simulink model "SinglePhasePVGridConnettedArray"  (R2024a)
settings: Solver=VariableStepAuto  StartTime=0.0  StopTime=0.1  RelTol=1e-3
libraries: spsMosfetLib x12, spsSeriesRLCBranchLib x12, spsCurrentMeasurementLib x6, spsFirstOrderFilterLib x6, slpidlib x6, simulink x6, spsVoltageMeasurementLib x6, spsACVoltageSourceLib x3, spsAlphaBetaZerotodq0Lib x3, spsPVArrayLib x3, spspowerguiLib x3
settings Model: Creator=Akbar  LastModifiedBy=Akbar
settings OptimizationCC: ReuseModelBlockBuffer=off
settings RTWCC: GPUComputeCapability=3.5

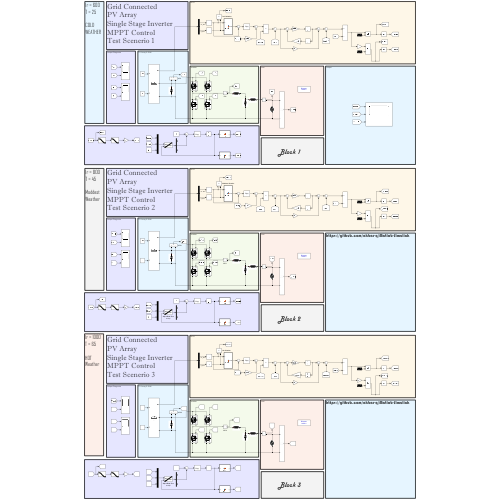
[thumbnail: Simulink's stored preview of the top-level diagram]
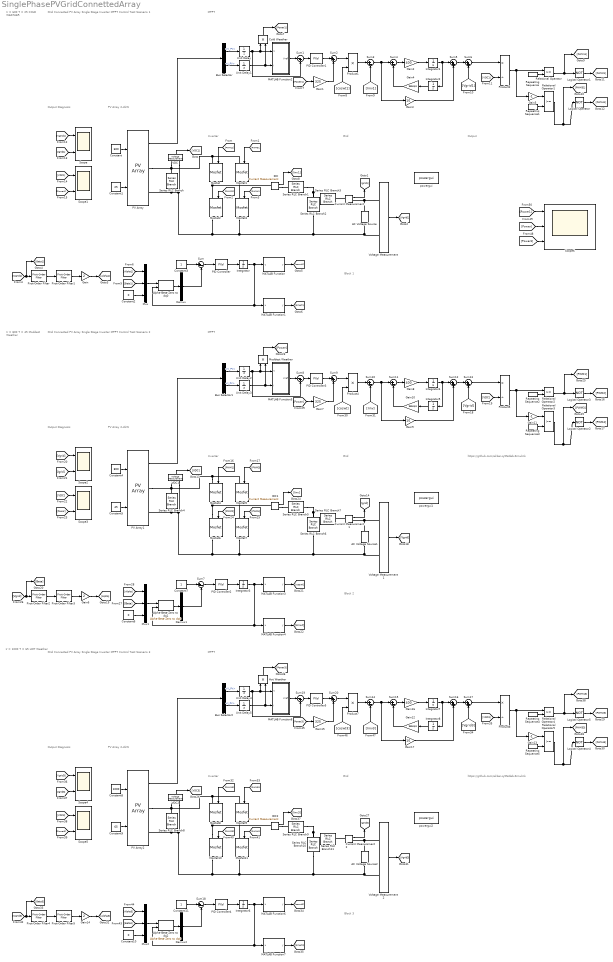
== system SinglePhasePVGridConnettedArray ==
  note: Output
  note: Ir = 600
      | T = 25
      |
      | COLD
      | WEATHER
  note: Grid Connected
      | PV Array
      | Single Stage Inverter
      | MPPT Control
      | Test Scenerio 1
  note: Block 1
  note: Grid
  note: Inverter
  note: PV Array 2-3kW
  note: MPPT
  note: Output Diagnosis
  note: Ir = 800
      | T = 45
      |
      | Moddest
      | Weather
  note: Grid Connected
      | PV Array
      | Single Stage Inverter
      | MPPT Control
      | Test Scenerio 2
  note: Inverter
  note: Grid
  note: PV Array 2-3kW
  note: Block 2
  note: Output Diagnosis
  note: MPPT
  note: Block 3
  note: PV Array 2-3kW
  note: Grid
  note: MPPT
  note: Output Diagnosis
  note: Ir = 1000
      | T = 65
      |
      | HOT
      | Weather
  note: Inverter
  note: Grid Connected
      | PV Array
      | Single Stage Inverter
      | MPPT Control
      | Test Scenerio 3
  note: https://github.com/akbar-q/Matlab-Simulink
  note: https://github.com/akbar-q/Matlab-Simulink
  AC Voltage Source : spsACVoltageSourceLib/AC Voltage Source  Amplitude=325  Phase=0  Frequency=50  SampleTime=0  Measurements=None  BusType=swing  Pref=10e3  Qref=0  Qmin=-inf  Qmax=+inf
  AC Voltage Source1 : spsACVoltageSourceLib/AC Voltage Source  Amplitude=325  Phase=0  Frequency=50  SampleTime=0  Measurements=None  BusType=swing  Pref=10e3  Qref=0  Qmin=-inf  Qmax=+inf
  AC Voltage Source2 : spsACVoltageSourceLib/AC Voltage Source  Amplitude=325  Phase=0  Frequency=50  SampleTime=0  Measurements=None  BusType=swing  Pref=10e3  Qref=0  Qmin=-inf  Qmax=+inf
  Alpha-Beta-Zero to dq0 : spsAlphaBetaZerotodq0Lib/Alpha-Beta-Zero to dq0  Alignment=90 degrees behind phase A axis
  Alpha-Beta-Zero to dq1 : spsAlphaBetaZerotodq0Lib/Alpha-Beta-Zero to dq0  Alignment=90 degrees behind phase A axis
  Alpha-Beta-Zero to dq2 : spsAlphaBetaZerotodq0Lib/Alpha-Beta-Zero to dq0  Alignment=90 degrees behind phase A axis
  Bus Selector : BusSelector  OutputSignals=V_PV,I_PV
  Bus Selector1 : BusSelector  OutputSignals=V_PV,I_PV
  Bus Selector2 : BusSelector  OutputSignals=V_PV,I_PV
  Cold Weather : Product
  Constant : Constant  Value=600
  Constant1 : Constant  Value=25
  Constant10 : Constant  Value=0
  Constant11 : Constant
  Constant2 : Constant  Value=0
  Constant3 : Constant
  Constant4 : Constant  Value=800
  Constant5 : Constant  Value=45
  Constant6 : Constant  Value=0
  Constant7 : Constant
  Constant8 : Constant  Value=1000
  Constant9 : Constant  Value=65
  Current Measurement : spsCurrentMeasurementLib/Current Measurement  PhasorSimulation=off  OutputType=Complex  PSBequivalent=0
  Current Measurement1 : spsCurrentMeasurementLib/Current Measurement  PhasorSimulation=off  OutputType=Complex  PSBequivalent=0
  Current Measurement2 : spsCurrentMeasurementLib/Current Measurement  PhasorSimulation=off  OutputType=Complex  PSBequivalent=0
  Demux : Demux  Outputs=3
  Demux1 : Demux  Outputs=3
  Demux2 : Demux  Outputs=3
  First-Order Filter{,1..5} (6 alike) : spsFirstOrderFilterLib/First-Order Filter  FilterType=Lowpass  Tc=1/(2*pi*50)  Ts=0  Initialize=off  Vac_Init=[0, 0, 60]  Vdc_Init=0  PlotResponse=off  FreqRange="[0,  200,  1]"
  Gain : Gain  Gain=2
  Gain1 : Gain  Gain=325
  Gain10 : Gain  Gain=986.8/4
  Gain11 : Gain  Gain=-1
  Gain12 : Gain  Gain=986.8/4
  Gain13 : Gain  Gain=-1
  Gain14 : Gain  Gain=2
  Gain15 : Gain  Gain=325
  Gain16 : Gain  Gain=400
  Gain17 : Gain  Gain=10
  Gain2 : Gain  Gain=400
  Gain3 : Gain  Gain=10
  Gain4 : Gain  Gain=986.8/4
  Gain5 : Gain  Gain=-1
  Gain6 : Gain  Gain=2
  Gain7 : Gain  Gain=325
  Gain8 : Gain  Gain=400
  Gain9 : Gain  Gain=10
  Hot Weather : Product
  IDC : spsCurrentMeasurementLib/Current Measurement  PhasorSimulation=off  OutputType=Complex  PSBequivalent=0
  IDC1 : spsCurrentMeasurementLib/Current Measurement  PhasorSimulation=off  OutputType=Complex  PSBequivalent=0
  IDC2 : spsCurrentMeasurementLib/Current Measurement  PhasorSimulation=off  OutputType=Complex  PSBequivalent=0
  Integrator{,1..8} (9 alike) : Integrator
  Logical Operator{,1..5} (6 alike) : Logic  Operator=NOT  AllPortsSameDT=off  OutDataTypeStr=boolean
  MATLAB Function : MATLAB Function  TreatAsAtomicUnit=on
  MATLAB Function1 : MATLAB Function  TreatAsAtomicUnit=on
  MATLAB Function2 : MATLAB Function  TreatAsAtomicUnit=on
  MATLAB Function3 : MATLAB Function  TreatAsAtomicUnit=on
  MATLAB Function4 : MATLAB Function  TreatAsAtomicUnit=on
  MATLAB Function5 : MATLAB Function  TreatAsAtomicUnit=on
  MATLAB Function6 : MATLAB Function  TreatAsAtomicUnit=on
  MATLAB Function7 : MATLAB Function  TreatAsAtomicUnit=on
  MATLAB Function8 : MATLAB Function  TreatAsAtomicUnit=on
  Moddest Weather : Product
  Mosfet{,1..11} (12 alike) : spsMosfetLib/Mosfet  Ron=0.1  Lon=0  Rd=0.01  Vfd=0  IC=0  Rs=1e5  Cs=inf  Measurements=on
  Mux : Mux  Inputs=3
  Mux1 : Mux  Inputs=3
  Mux2 : Mux  Inputs=3
  PID Controller : slpidlib/PID Controller  Controller=PI  Form=Parallel  TimeDomain=Continuous-time  UseExternalTs=off  SampleTime=-1  IntegratorMethod=Forward Euler  FilterMethod=Forward Euler  ControllerParametersSource=internal  P=10  I=5000  UseKiTs=off  D=0  UseExternalDerivativeSource=off  N=100  UseFilter=on  TunerSelectOption=Transfer Function Based (PID Tuner App)  InitialConditionSource=internal  InitialConditionForIntegrator=0  InitialConditionForFilter=0  DifferentiatorICPrevScaledInput=0  ExternalReset=none  TrackingMode=off  Kt=1  LimitOutput=off  SatLimitsSource=internal  UpperSaturationLimit=inf  LowerSaturationLimit=-inf  LinearizeAsGain=on  AntiWindupMode=none  Kb=1  LimitIntegrator=off  UpperIntegratorSaturationLimit=inf  LowerIntegratorSaturationLimit=-inf  POutMin=[]  POutMax=[]  IOutMin=[]  IOutMax=[]  DOutMin=[]  DOutMax=[]  NOutMin=[]  NOutMax=[]  SumOutMin=[]  SumOutMax=[]  SaturationOutMin=[]  SaturationOutMax=[]  PParamMin=[]  PParamMax=[]  IParamMin=[]  IParamMax=[]  DParamMin=[]  DParamMax=[]  NParamMin=[]  NParamMax=[]  KbParamMin=[]  KbParamMax=[]  KtParamMin=[]  KtParamMax=[]  KbOutMin=[]  KbOutMax=[]  KtOutMin=[]  KtOutMax=[]  IntegratorOutMin=[]  IntegratorOutMax=[]  FilterOutMin=[]  FilterOutMax=[]  SumI1OutMin=[]  SumI1OutMax=[]  SumI2OutMin=[]  SumI2OutMax=[]  SumI3OutMin=[]  SumI3OutMax=[]  SumI4OutMin=[]  SumI4OutMax=[]  SumDOutMin=[]  SumDOutMax=[]  DifferentiatorOutMin=[]  DifferentiatorOutMax=[]  FilterDiffOutCoefMin=[]  FilterDiffOutCoefMax=[]  ReciprocalOutMin=[]  ReciprocalOutMax=[]  SumDenOutMin=[]  SumDenOutMax=[]  SumNumOutMin=[]  SumNumOutMax=[]  DivideOutMin=[]  DivideOutMax=[]  UdiffTsProdOutMin=[]  UdiffTsProdOutMax=[]  NTsProdOutMin=[]  NTsProdOutMax=[]  UintegralTsProdOutMin=[]  UintegralTsProdOutMax=[]  UngainTsProdOutMin=[]  UngainTsProdOutMax=[]  ClampingZeroOutDataTypeStr=Inherit: Inherit via back propagation  ClampingZeroOutMin=[]  ClampingZeroOutMax=[]  FilterDenConstantOutDataTypeStr=Inherit: Inherit via back propagation  FilterDenConstantOutMin=[]  FilterDenConstantOutMax=[]  PCopyOutDataTypeStr=Inherit: Inherit via back propagation  PCopyOutMin=[]  PCopyOutMax=[]  NCopyOutDataTypeStr=Inherit: Inherit via back propagation  NCopyOutMin=[]  NCopyOutMax=[]  IntegratorContinuousStateAttributes=''  IntegratorStateMustResolveToSignalObject=off  IntegratorRTWStateStorageClass=Auto  FilterContinuousStateAttributes=''  FilterStateMustResolveToSignalObject=off  FilterRTWStateStorageClass=Auto  ParallelPVariant=InternalParameters  IdealPVariant=Disabled  IVariant=InternalParameters  DVariant=Disabled  IntegratorVariant=Continuous  SatVariant=Disabled  AWVariant=Passthrough  PCopyVariant=Disabled  TRVariant=Disabled  FdbkBlocksVariant=Forward  IdealPFdbkVariant=Disabled  SatFdbkVariant=Disabled  DerivativeFilterVariant=Disabled  NVariant=Disabled  NCopyVariant=Disabled_SignalSpec  FilterICVariant=Disabled  IntegratorICVariant=InternalICs  ExternalResetVariant=Disabled  TRSumVariant=Passthrough  SumFdbkVariant=Disabled  SumVariant=Sum_PI  TsampFilterVariant=InternalTs  TsampNgainVariant=Passthrough  TsampIntegralVariant=Disabled_SignalSpec  ExternalSaturationOutDataTypeStr=Inherit: Same as second input  DerivativeSourceVariant=Disabled
  PID Controller1 : slpidlib/PID Controller  Controller=PI  Form=Parallel  TimeDomain=Continuous-time  UseExternalTs=off  SampleTime=-1  IntegratorMethod=Forward Euler  FilterMethod=Forward Euler  ControllerParametersSource=internal  P=0.075  I=0.075  UseKiTs=off  D=0  UseExternalDerivativeSource=off  N=100  UseFilter=on  TunerSelectOption=Transfer Function Based (PID Tuner App)  InitialConditionSource=internal  InitialConditionForIntegrator=0  InitialConditionForFilter=0  DifferentiatorICPrevScaledInput=0  ExternalReset=none  TrackingMode=off  Kt=1  LimitOutput=off  SatLimitsSource=internal  UpperSaturationLimit=inf  LowerSaturationLimit=-inf  LinearizeAsGain=on  AntiWindupMode=none  Kb=1  LimitIntegrator=off  UpperIntegratorSaturationLimit=inf  LowerIntegratorSaturationLimit=-inf  POutMin=[]  POutMax=[]  IOutMin=[]  IOutMax=[]  DOutMin=[]  DOutMax=[]  NOutMin=[]  NOutMax=[]  SumOutMin=[]  SumOutMax=[]  SaturationOutMin=[]  SaturationOutMax=[]  PParamMin=[]  PParamMax=[]  IParamMin=[]  IParamMax=[]  DParamMin=[]  DParamMax=[]  NParamMin=[]  NParamMax=[]  KbParamMin=[]  KbParamMax=[]  KtParamMin=[]  KtParamMax=[]  KbOutMin=[]  KbOutMax=[]  KtOutMin=[]  KtOutMax=[]  IntegratorOutMin=[]  IntegratorOutMax=[]  FilterOutMin=[]  FilterOutMax=[]  SumI1OutMin=[]  SumI1OutMax=[]  SumI2OutMin=[]  SumI2OutMax=[]  SumI3OutMin=[]  SumI3OutMax=[]  SumI4OutMin=[]  SumI4OutMax=[]  SumDOutMin=[]  SumDOutMax=[]  DifferentiatorOutMin=[]  DifferentiatorOutMax=[]  FilterDiffOutCoefMin=[]  FilterDiffOutCoefMax=[]  ReciprocalOutMin=[]  ReciprocalOutMax=[]  SumDenOutMin=[]  SumDenOutMax=[]  SumNumOutMin=[]  SumNumOutMax=[]  DivideOutMin=[]  DivideOutMax=[]  UdiffTsProdOutMin=[]  UdiffTsProdOutMax=[]  NTsProdOutMin=[]  NTsProdOutMax=[]  UintegralTsProdOutMin=[]  UintegralTsProdOutMax=[]  UngainTsProdOutMin=[]  UngainTsProdOutMax=[]  ClampingZeroOutDataTypeStr=Inherit: Inherit via back propagation  ClampingZeroOutMin=[]  ClampingZeroOutMax=[]  FilterDenConstantOutDataTypeStr=Inherit: Inherit via back propagation  FilterDenConstantOutMin=[]  FilterDenConstantOutMax=[]  PCopyOutDataTypeStr=Inherit: Inherit via back propagation  PCopyOutMin=[]  PCopyOutMax=[]  NCopyOutDataTypeStr=Inherit: Inherit via back propagation  NCopyOutMin=[]  NCopyOutMax=[]  IntegratorContinuousStateAttributes=''  IntegratorStateMustResolveToSignalObject=off  IntegratorRTWStateStorageClass=Auto  FilterContinuousStateAttributes=''  FilterStateMustResolveToSignalObject=off  FilterRTWStateStorageClass=Auto  ParallelPVariant=InternalParameters  IdealPVariant=Disabled  IVariant=InternalParameters  DVariant=Disabled  IntegratorVariant=Continuous  SatVariant=Disabled  AWVariant=Passthrough  PCopyVariant=Disabled  TRVariant=Disabled  FdbkBlocksVariant=Forward  IdealPFdbkVariant=Disabled  SatFdbkVariant=Disabled  DerivativeFilterVariant=Disabled  NVariant=Disabled  NCopyVariant=Disabled_SignalSpec  FilterICVariant=Disabled  IntegratorICVariant=InternalICs  ExternalResetVariant=Disabled  TRSumVariant=Passthrough  SumFdbkVariant=Disabled  SumVariant=Sum_PI  TsampFilterVariant=InternalTs  TsampNgainVariant=Passthrough  TsampIntegralVariant=Disabled_SignalSpec  ExternalSaturationOutDataTypeStr=Inherit: Same as second input  DerivativeSourceVariant=Disabled
  PID Controller2 : slpidlib/PID Controller  Controller=PI  Form=Parallel  TimeDomain=Continuous-time  UseExternalTs=off  SampleTime=-1  IntegratorMethod=Forward Euler  FilterMethod=Forward Euler  ControllerParametersSource=internal  P=10  I=5000  UseKiTs=off  D=0  UseExternalDerivativeSource=off  N=100  UseFilter=on  TunerSelectOption=Transfer Function Based (PID Tuner App)  InitialConditionSource=internal  InitialConditionForIntegrator=0  InitialConditionForFilter=0  DifferentiatorICPrevScaledInput=0  ExternalReset=none  TrackingMode=off  Kt=1  LimitOutput=off  SatLimitsSource=internal  UpperSaturationLimit=inf  LowerSaturationLimit=-inf  LinearizeAsGain=on  AntiWindupMode=none  Kb=1  LimitIntegrator=off  UpperIntegratorSaturationLimit=inf  LowerIntegratorSaturationLimit=-inf  POutMin=[]  POutMax=[]  IOutMin=[]  IOutMax=[]  DOutMin=[]  DOutMax=[]  NOutMin=[]  NOutMax=[]  SumOutMin=[]  SumOutMax=[]  SaturationOutMin=[]  SaturationOutMax=[]  PParamMin=[]  PParamMax=[]  IParamMin=[]  IParamMax=[]  DParamMin=[]  DParamMax=[]  NParamMin=[]  NParamMax=[]  KbParamMin=[]  KbParamMax=[]  KtParamMin=[]  KtParamMax=[]  KbOutMin=[]  KbOutMax=[]  KtOutMin=[]  KtOutMax=[]  IntegratorOutMin=[]  IntegratorOutMax=[]  FilterOutMin=[]  FilterOutMax=[]  SumI1OutMin=[]  SumI1OutMax=[]  SumI2OutMin=[]  SumI2OutMax=[]  SumI3OutMin=[]  SumI3OutMax=[]  SumI4OutMin=[]  SumI4OutMax=[]  SumDOutMin=[]  SumDOutMax=[]  DifferentiatorOutMin=[]  DifferentiatorOutMax=[]  FilterDiffOutCoefMin=[]  FilterDiffOutCoefMax=[]  ReciprocalOutMin=[]  ReciprocalOutMax=[]  SumDenOutMin=[]  SumDenOutMax=[]  SumNumOutMin=[]  SumNumOutMax=[]  DivideOutMin=[]  DivideOutMax=[]  UdiffTsProdOutMin=[]  UdiffTsProdOutMax=[]  NTsProdOutMin=[]  NTsProdOutMax=[]  UintegralTsProdOutMin=[]  UintegralTsProdOutMax=[]  UngainTsProdOutMin=[]  UngainTsProdOutMax=[]  ClampingZeroOutDataTypeStr=Inherit: Inherit via back propagation  ClampingZeroOutMin=[]  ClampingZeroOutMax=[]  FilterDenConstantOutDataTypeStr=Inherit: Inherit via back propagation  FilterDenConstantOutMin=[]  FilterDenConstantOutMax=[]  PCopyOutDataTypeStr=Inherit: Inherit via back propagation  PCopyOutMin=[]  PCopyOutMax=[]  NCopyOutDataTypeStr=Inherit: Inherit via back propagation  NCopyOutMin=[]  NCopyOutMax=[]  IntegratorContinuousStateAttributes=''  IntegratorStateMustResolveToSignalObject=off  IntegratorRTWStateStorageClass=Auto  FilterContinuousStateAttributes=''  FilterStateMustResolveToSignalObject=off  FilterRTWStateStorageClass=Auto  ParallelPVariant=InternalParameters  IdealPVariant=Disabled  IVariant=InternalParameters  DVariant=Disabled  IntegratorVariant=Continuous  SatVariant=Disabled  AWVariant=Passthrough  PCopyVariant=Disabled  TRVariant=Disabled  FdbkBlocksVariant=Forward  IdealPFdbkVariant=Disabled  SatFdbkVariant=Disabled  DerivativeFilterVariant=Disabled  NVariant=Disabled  NCopyVariant=Disabled_SignalSpec  FilterICVariant=Disabled  IntegratorICVariant=InternalICs  ExternalResetVariant=Disabled  TRSumVariant=Passthrough  SumFdbkVariant=Disabled  SumVariant=Sum_PI  TsampFilterVariant=InternalTs  TsampNgainVariant=Passthrough  TsampIntegralVariant=Disabled_SignalSpec  ExternalSaturationOutDataTypeStr=Inherit: Same as second input  DerivativeSourceVariant=Disabled
  PID Controller3 : slpidlib/PID Controller  Controller=PI  Form=Parallel  TimeDomain=Continuous-time  UseExternalTs=off  SampleTime=-1  IntegratorMethod=Forward Euler  FilterMethod=Forward Euler  ControllerParametersSource=internal  P=0.075  I=0.075  UseKiTs=off  D=0  UseExternalDerivativeSource=off  N=100  UseFilter=on  TunerSelectOption=Transfer Function Based (PID Tuner App)  InitialConditionSource=internal  InitialConditionForIntegrator=0  InitialConditionForFilter=0  DifferentiatorICPrevScaledInput=0  ExternalReset=none  TrackingMode=off  Kt=1  LimitOutput=off  SatLimitsSource=internal  UpperSaturationLimit=inf  LowerSaturationLimit=-inf  LinearizeAsGain=on  AntiWindupMode=none  Kb=1  LimitIntegrator=off  UpperIntegratorSaturationLimit=inf  LowerIntegratorSaturationLimit=-inf  POutMin=[]  POutMax=[]  IOutMin=[]  IOutMax=[]  DOutMin=[]  DOutMax=[]  NOutMin=[]  NOutMax=[]  SumOutMin=[]  SumOutMax=[]  SaturationOutMin=[]  SaturationOutMax=[]  PParamMin=[]  PParamMax=[]  IParamMin=[]  IParamMax=[]  DParamMin=[]  DParamMax=[]  NParamMin=[]  NParamMax=[]  KbParamMin=[]  KbParamMax=[]  KtParamMin=[]  KtParamMax=[]  KbOutMin=[]  KbOutMax=[]  KtOutMin=[]  KtOutMax=[]  IntegratorOutMin=[]  IntegratorOutMax=[]  FilterOutMin=[]  FilterOutMax=[]  SumI1OutMin=[]  SumI1OutMax=[]  SumI2OutMin=[]  SumI2OutMax=[]  SumI3OutMin=[]  SumI3OutMax=[]  SumI4OutMin=[]  SumI4OutMax=[]  SumDOutMin=[]  SumDOutMax=[]  DifferentiatorOutMin=[]  DifferentiatorOutMax=[]  FilterDiffOutCoefMin=[]  FilterDiffOutCoefMax=[]  ReciprocalOutMin=[]  ReciprocalOutMax=[]  SumDenOutMin=[]  SumDenOutMax=[]  SumNumOutMin=[]  SumNumOutMax=[]  DivideOutMin=[]  DivideOutMax=[]  UdiffTsProdOutMin=[]  UdiffTsProdOutMax=[]  NTsProdOutMin=[]  NTsProdOutMax=[]  UintegralTsProdOutMin=[]  UintegralTsProdOutMax=[]  UngainTsProdOutMin=[]  UngainTsProdOutMax=[]  ClampingZeroOutDataTypeStr=Inherit: Inherit via back propagation  ClampingZeroOutMin=[]  ClampingZeroOutMax=[]  FilterDenConstantOutDataTypeStr=Inherit: Inherit via back propagation  FilterDenConstantOutMin=[]  FilterDenConstantOutMax=[]  PCopyOutDataTypeStr=Inherit: Inherit via back propagation  PCopyOutMin=[]  PCopyOutMax=[]  NCopyOutDataTypeStr=Inherit: Inherit via back propagation  NCopyOutMin=[]  NCopyOutMax=[]  IntegratorContinuousStateAttributes=''  IntegratorStateMustResolveToSignalObject=off  IntegratorRTWStateStorageClass=Auto  FilterContinuousStateAttributes=''  FilterStateMustResolveToSignalObject=off  FilterRTWStateStorageClass=Auto  ParallelPVariant=InternalParameters  IdealPVariant=Disabled  IVariant=InternalParameters  DVariant=Disabled  IntegratorVariant=Continuous  SatVariant=Disabled  AWVariant=Passthrough  PCopyVariant=Disabled  TRVariant=Disabled  FdbkBlocksVariant=Forward  IdealPFdbkVariant=Disabled  SatFdbkVariant=Disabled  DerivativeFilterVariant=Disabled  NVariant=Disabled  NCopyVariant=Disabled_SignalSpec  FilterICVariant=Disabled  IntegratorICVariant=InternalICs  ExternalResetVariant=Disabled  TRSumVariant=Passthrough  SumFdbkVariant=Disabled  SumVariant=Sum_PI  TsampFilterVariant=InternalTs  TsampNgainVariant=Passthrough  TsampIntegralVariant=Disabled_SignalSpec  ExternalSaturationOutDataTypeStr=Inherit: Same as second input  DerivativeSourceVariant=Disabled
  PID Controller4 : slpidlib/PID Controller  Controller=PI  Form=Parallel  TimeDomain=Continuous-time  UseExternalTs=off  SampleTime=-1  IntegratorMethod=Forward Euler  FilterMethod=Forward Euler  ControllerParametersSource=internal  P=10  I=5000  UseKiTs=off  D=0  UseExternalDerivativeSource=off  N=100  UseFilter=on  TunerSelectOption=Transfer Function Based (PID Tuner App)  InitialConditionSource=internal  InitialConditionForIntegrator=0  InitialConditionForFilter=0  DifferentiatorICPrevScaledInput=0  ExternalReset=none  TrackingMode=off  Kt=1  LimitOutput=off  SatLimitsSource=internal  UpperSaturationLimit=inf  LowerSaturationLimit=-inf  LinearizeAsGain=on  AntiWindupMode=none  Kb=1  LimitIntegrator=off  UpperIntegratorSaturationLimit=inf  LowerIntegratorSaturationLimit=-inf  POutMin=[]  POutMax=[]  IOutMin=[]  IOutMax=[]  DOutMin=[]  DOutMax=[]  NOutMin=[]  NOutMax=[]  SumOutMin=[]  SumOutMax=[]  SaturationOutMin=[]  SaturationOutMax=[]  PParamMin=[]  PParamMax=[]  IParamMin=[]  IParamMax=[]  DParamMin=[]  DParamMax=[]  NParamMin=[]  NParamMax=[]  KbParamMin=[]  KbParamMax=[]  KtParamMin=[]  KtParamMax=[]  KbOutMin=[]  KbOutMax=[]  KtOutMin=[]  KtOutMax=[]  IntegratorOutMin=[]  IntegratorOutMax=[]  FilterOutMin=[]  FilterOutMax=[]  SumI1OutMin=[]  SumI1OutMax=[]  SumI2OutMin=[]  SumI2OutMax=[]  SumI3OutMin=[]  SumI3OutMax=[]  SumI4OutMin=[]  SumI4OutMax=[]  SumDOutMin=[]  SumDOutMax=[]  DifferentiatorOutMin=[]  DifferentiatorOutMax=[]  FilterDiffOutCoefMin=[]  FilterDiffOutCoefMax=[]  ReciprocalOutMin=[]  ReciprocalOutMax=[]  SumDenOutMin=[]  SumDenOutMax=[]  SumNumOutMin=[]  SumNumOutMax=[]  DivideOutMin=[]  DivideOutMax=[]  UdiffTsProdOutMin=[]  UdiffTsProdOutMax=[]  NTsProdOutMin=[]  NTsProdOutMax=[]  UintegralTsProdOutMin=[]  UintegralTsProdOutMax=[]  UngainTsProdOutMin=[]  UngainTsProdOutMax=[]  ClampingZeroOutDataTypeStr=Inherit: Inherit via back propagation  ClampingZeroOutMin=[]  ClampingZeroOutMax=[]  FilterDenConstantOutDataTypeStr=Inherit: Inherit via back propagation  FilterDenConstantOutMin=[]  FilterDenConstantOutMax=[]  PCopyOutDataTypeStr=Inherit: Inherit via back propagation  PCopyOutMin=[]  PCopyOutMax=[]  NCopyOutDataTypeStr=Inherit: Inherit via back propagation  NCopyOutMin=[]  NCopyOutMax=[]  IntegratorContinuousStateAttributes=''  IntegratorStateMustResolveToSignalObject=off  IntegratorRTWStateStorageClass=Auto  FilterContinuousStateAttributes=''  FilterStateMustResolveToSignalObject=off  FilterRTWStateStorageClass=Auto  ParallelPVariant=InternalParameters  IdealPVariant=Disabled  IVariant=InternalParameters  DVariant=Disabled  IntegratorVariant=Continuous  SatVariant=Disabled  AWVariant=Passthrough  PCopyVariant=Disabled  TRVariant=Disabled  FdbkBlocksVariant=Forward  IdealPFdbkVariant=Disabled  SatFdbkVariant=Disabled  DerivativeFilterVariant=Disabled  NVariant=Disabled  NCopyVariant=Disabled_SignalSpec  FilterICVariant=Disabled  IntegratorICVariant=InternalICs  ExternalResetVariant=Disabled  TRSumVariant=Passthrough  SumFdbkVariant=Disabled  SumVariant=Sum_PI  TsampFilterVariant=InternalTs  TsampNgainVariant=Passthrough  TsampIntegralVariant=Disabled_SignalSpec  ExternalSaturationOutDataTypeStr=Inherit: Same as second input  DerivativeSourceVariant=Disabled
  PID Controller5 : slpidlib/PID Controller  Controller=PI  Form=Parallel  TimeDomain=Continuous-time  UseExternalTs=off  SampleTime=-1  IntegratorMethod=Forward Euler  FilterMethod=Forward Euler  ControllerParametersSource=internal  P=0.075  I=0.075  UseKiTs=off  D=0  UseExternalDerivativeSource=off  N=100  UseFilter=on  TunerSelectOption=Transfer Function Based (PID Tuner App)  InitialConditionSource=internal  InitialConditionForIntegrator=0  InitialConditionForFilter=0  DifferentiatorICPrevScaledInput=0  ExternalReset=none  TrackingMode=off  Kt=1  LimitOutput=off  SatLimitsSource=internal  UpperSaturationLimit=inf  LowerSaturationLimit=-inf  LinearizeAsGain=on  AntiWindupMode=none  Kb=1  LimitIntegrator=off  UpperIntegratorSaturationLimit=inf  LowerIntegratorSaturationLimit=-inf  POutMin=[]  POutMax=[]  IOutMin=[]  IOutMax=[]  DOutMin=[]  DOutMax=[]  NOutMin=[]  NOutMax=[]  SumOutMin=[]  SumOutMax=[]  SaturationOutMin=[]  SaturationOutMax=[]  PParamMin=[]  PParamMax=[]  IParamMin=[]  IParamMax=[]  DParamMin=[]  DParamMax=[]  NParamMin=[]  NParamMax=[]  KbParamMin=[]  KbParamMax=[]  KtParamMin=[]  KtParamMax=[]  KbOutMin=[]  KbOutMax=[]  KtOutMin=[]  KtOutMax=[]  IntegratorOutMin=[]  IntegratorOutMax=[]  FilterOutMin=[]  FilterOutMax=[]  SumI1OutMin=[]  SumI1OutMax=[]  SumI2OutMin=[]  SumI2OutMax=[]  SumI3OutMin=[]  SumI3OutMax=[]  SumI4OutMin=[]  SumI4OutMax=[]  SumDOutMin=[]  SumDOutMax=[]  DifferentiatorOutMin=[]  DifferentiatorOutMax=[]  FilterDiffOutCoefMin=[]  FilterDiffOutCoefMax=[]  ReciprocalOutMin=[]  ReciprocalOutMax=[]  SumDenOutMin=[]  SumDenOutMax=[]  SumNumOutMin=[]  SumNumOutMax=[]  DivideOutMin=[]  DivideOutMax=[]  UdiffTsProdOutMin=[]  UdiffTsProdOutMax=[]  NTsProdOutMin=[]  NTsProdOutMax=[]  UintegralTsProdOutMin=[]  UintegralTsProdOutMax=[]  UngainTsProdOutMin=[]  UngainTsProdOutMax=[]  ClampingZeroOutDataTypeStr=Inherit: Inherit via back propagation  ClampingZeroOutMin=[]  ClampingZeroOutMax=[]  FilterDenConstantOutDataTypeStr=Inherit: Inherit via back propagation  FilterDenConstantOutMin=[]  FilterDenConstantOutMax=[]  PCopyOutDataTypeStr=Inherit: Inherit via back propagation  PCopyOutMin=[]  PCopyOutMax=[]  NCopyOutDataTypeStr=Inherit: Inherit via back propagation  NCopyOutMin=[]  NCopyOutMax=[]  IntegratorContinuousStateAttributes=''  IntegratorStateMustResolveToSignalObject=off  IntegratorRTWStateStorageClass=Auto  FilterContinuousStateAttributes=''  FilterStateMustResolveToSignalObject=off  FilterRTWStateStorageClass=Auto  ParallelPVariant=InternalParameters  IdealPVariant=Disabled  IVariant=InternalParameters  DVariant=Disabled  IntegratorVariant=Continuous  SatVariant=Disabled  AWVariant=Passthrough  PCopyVariant=Disabled  TRVariant=Disabled  FdbkBlocksVariant=Forward  IdealPFdbkVariant=Disabled  SatFdbkVariant=Disabled  DerivativeFilterVariant=Disabled  NVariant=Disabled  NCopyVariant=Disabled_SignalSpec  FilterICVariant=Disabled  IntegratorICVariant=InternalICs  ExternalResetVariant=Disabled  TRSumVariant=Passthrough  SumFdbkVariant=Disabled  SumVariant=Sum_PI  TsampFilterVariant=InternalTs  TsampNgainVariant=Passthrough  TsampIntegralVariant=Disabled_SignalSpec  ExternalSaturationOutDataTypeStr=Inherit: Same as second input  DerivativeSourceVariant=Disabled
  PV Array : spsPVArrayLib/PV Array  Npar=1  Nser=14  PlotType=array @ 1000 W/m2 & specified temperatures  S_vec="[ 1000  500  100 ]"  Temp_C_vec="[ 45 25  ]"  ModuleName=A2Peak Power POWER ON P220-6x10  PlotWhenSelected=off  Pm=219.978  Ncell=60  Voc=36.72  Isc=7.98  Vm=30.3  Im=7.26  beta_Voc_pc=-0.35  alpha_Isc_pc=0.05  beta_Voc=-0.12852  alpha_Isc=0.00399  IL=8.0041  I0=1.8441e-10  nI=0.97472  Rsh=85.0716  Rs=0.25728  RobustModel=off  RobustCellTemperature=313.3991  BAL=on  Tc=1e-6  Tfilter=5e-5
  PV Array1 : spsPVArrayLib/PV Array  Npar=1  Nser=14  PlotType=array @ 1000 W/m2 & specified temperatures  S_vec="[ 1000  500  100 ]"  Temp_C_vec="[ 45 25  ]"  ModuleName=A2Peak Power POWER ON P220-6x10  PlotWhenSelected=off  Pm=219.978  Ncell=60  Voc=36.72  Isc=7.98  Vm=30.3  Im=7.26  beta_Voc_pc=-0.35  alpha_Isc_pc=0.05  beta_Voc=-0.12852  alpha_Isc=0.00399  IL=8.0041  I0=1.8441e-10  nI=0.97472  Rsh=85.0716  Rs=0.25728  RobustModel=off  RobustCellTemperature=313.3991  BAL=on  Tc=1e-6  Tfilter=5e-5
  PV Array2 : spsPVArrayLib/PV Array  Npar=1  Nser=14  PlotType=array @ 1000 W/m2 & specified temperatures  S_vec="[ 1000  500  100 ]"  Temp_C_vec="[ 45 25  ]"  ModuleName=A2Peak Power POWER ON P220-6x10  PlotWhenSelected=off  Pm=219.978  Ncell=60  Voc=36.72  Isc=7.98  Vm=30.3  Im=7.26  beta_Voc_pc=-0.35  alpha_Isc_pc=0.05  beta_Voc=-0.12852  alpha_Isc=0.00399  IL=8.0041  I0=1.8441e-10  nI=0.97472  Rsh=85.0716  Rs=0.25728  RobustModel=off  RobustCellTemperature=313.3991  BAL=on  Tc=1e-6  Tfilter=5e-5
  Product1 : Product
  Product2 : Product  Inputs=*/
  Product4 : Product
  Product5 : Product  Inputs=*/
  Product7 : Product
  Product8 : Product  Inputs=*/
  Relational Operator{,1..5} (6 alike) : RelationalOperator  OutDataTypeStr=boolean  RndMeth=Simplest  InputSameDT=off
  Repeating Sequence{,1..5} (6 alike) : simulink/Sources/Repeating Sequence  rep_seq_t=[0 0.00005 0.0001]  rep_seq_y=[-1 1 -1]
  Scope{,1..5} (6 alike) : Scope  NumInputPorts=2
  Scope6 : Scope  NumInputPorts=3
  Series RLC Branch : spsSeriesRLCBranchLib/Series RLC Branch  LConnTagsString=__new0  RConnTagsString=__new0  BranchType=C  Resistance=1  Inductance=1e-3  SetiL0=off  InitialCurrent=0  Capacitance=600e-6  Setx0=on  InitialVoltage=470  Measurements=None
  Series RLC Branch1 : spsSeriesRLCBranchLib/Series RLC Branch  LConnTagsString=__new0  RConnTagsString=__new0  BranchType=L  Resistance=1  Inductance=4.06e-3  SetiL0=off  InitialCurrent=0  Capacitance=600e-6  Setx0=on  InitialVoltage=400  Measurements=None
  Series RLC Branch10 : spsSeriesRLCBranchLib/Series RLC Branch  LConnTagsString=__new0  RConnTagsString=__new0  BranchType=C  Resistance=1  Inductance=4.06e-3  SetiL0=off  InitialCurrent=0  Capacitance=6.23e-6  Setx0=on  InitialVoltage=400  Measurements=None
  Series RLC Branch11 : spsSeriesRLCBranchLib/Series RLC Branch  LConnTagsString=__new0  RConnTagsString=__new0  BranchType=L  Resistance=1  Inductance=4.35e-3  SetiL0=off  InitialCurrent=0  Capacitance=600e-6  Setx0=on  InitialVoltage=400  Measurements=None
  Series RLC Branch2 : spsSeriesRLCBranchLib/Series RLC Branch  LConnTagsString=__new0  RConnTagsString=__new0  BranchType=C  Resistance=1  Inductance=4.06e-3  SetiL0=off  InitialCurrent=0  Capacitance=6.23e-6  Setx0=on  InitialVoltage=400  Measurements=None
  Series RLC Branch3 : spsSeriesRLCBranchLib/Series RLC Branch  LConnTagsString=__new0  RConnTagsString=__new0  BranchType=L  Resistance=1  Inductance=4.35e-3  SetiL0=off  InitialCurrent=0  Capacitance=600e-6  Setx0=on  InitialVoltage=400  Measurements=None
  Series RLC Branch4 : spsSeriesRLCBranchLib/Series RLC Branch  LConnTagsString=__new0  RConnTagsString=__new0  BranchType=C  Resistance=1  Inductance=1e-3  SetiL0=off  InitialCurrent=0  Capacitance=600e-6  Setx0=on  InitialVoltage=470  Measurements=None
  Series RLC Branch5 : spsSeriesRLCBranchLib/Series RLC Branch  LConnTagsString=__new0  RConnTagsString=__new0  BranchType=L  Resistance=1  Inductance=4.06e-3  SetiL0=off  InitialCurrent=0  Capacitance=600e-6  Setx0=on  InitialVoltage=400  Measurements=None
  Series RLC Branch6 : spsSeriesRLCBranchLib/Series RLC Branch  LConnTagsString=__new0  RConnTagsString=__new0  BranchType=C  Resistance=1  Inductance=4.06e-3  SetiL0=off  InitialCurrent=0  Capacitance=6.23e-6  Setx0=on  InitialVoltage=400  Measurements=None
  Series RLC Branch7 : spsSeriesRLCBranchLib/Series RLC Branch  LConnTagsString=__new0  RConnTagsString=__new0  BranchType=L  Resistance=1  Inductance=4.35e-3  SetiL0=off  InitialCurrent=0  Capacitance=600e-6  Setx0=on  InitialVoltage=400  Measurements=None
  Series RLC Branch8 : spsSeriesRLCBranchLib/Series RLC Branch  LConnTagsString=__new0  RConnTagsString=__new0  BranchType=C  Resistance=1  Inductance=1e-3  SetiL0=off  InitialCurrent=0  Capacitance=600e-6  Setx0=on  InitialVoltage=470  Measurements=None
  Series RLC Branch9 : spsSeriesRLCBranchLib/Series RLC Branch  LConnTagsString=__new0  RConnTagsString=__new0  BranchType=L  Resistance=1  Inductance=4.06e-3  SetiL0=off  InitialCurrent=0  Capacitance=600e-6  Setx0=on  InitialVoltage=400  Measurements=None
  Sum{,3..4,7,10..11,14..15,18} (9 alike) : Sum  Inputs=|+-
  Sum1 : Sum  Inputs=|-+
  Sum{2,5..6,9,12..13,16..17,20} (9 alike) : Sum  Inputs=|++
  Sum19 : Sum  Inputs=|-+
  Sum8 : Sum  Inputs=|-+
  Unit Delay{,1..5} (6 alike) : UnitDelay  SampleTime=1e-4  HasFrameUpgradeWarning=on
  VDC : spsVoltageMeasurementLib/Voltage Measurement  PhasorSimulation=off  OutputType=Complex  PSBequivalent=0
  VDC1 : spsVoltageMeasurementLib/Voltage Measurement  PhasorSimulation=off  OutputType=Complex  PSBequivalent=0
  VDC2 : spsVoltageMeasurementLib/Voltage Measurement  PhasorSimulation=off  OutputType=Complex  PSBequivalent=0
  Voltage Measurement : spsVoltageMeasurementLib/Voltage Measurement  PhasorSimulation=off  OutputType=Complex  PSBequivalent=0
  Voltage Measurement1 : spsVoltageMeasurementLib/Voltage Measurement  PhasorSimulation=off  OutputType=Complex  PSBequivalent=0
  Voltage Measurement2 : spsVoltageMeasurementLib/Voltage Measurement  PhasorSimulation=off  OutputType=Complex  PSBequivalent=0
  powergui : spspowerguiLib/powergui  Priority=1  SimulationMode=Discrete  SampleTime=1e-6  frequency=60  Iterations=50  frequencyindice=50  Pbase=100e6  ErrMax=1e-4  UnitsV=kV  UnitsW=MW  buscounter=0  FunctionMessages=off  echomessages=off  EnableUseOfTLC=off  CurrentSourceSwitches=off  DisableSnubberDevices=off  DisableRonSwitches=off  DisableVfSwitches=off  DisplayEquations=off  AutomaticDiscreteSolvers=off  SolverType=Tustin/Backward Euler (TBE)  Interpol=off  ExternalGateDelay=off  methode=off  Ts=100  x0status=blocks  SPID=on  SwTol=0  HookPort=off  NonlinearTolerance=1e-4  nMaxIteration=100  ContinueOnMaxIteration=off  RestoreLinks=warning  ResistiveCurrentMeasurement=off  Frange=[0:2:500]  Ylog=off  Xlog=on  ShowGrid=off  save=off  variable=ZData  structure=0  ZoomFFT=off  StartTime=0.0  cycles=1  DisplayStyle=1  fundamental=60  FreqAxis=off  MaxFrequency=1000  frequencyindicesteady=1  RmsSteady=1  display=off
  powergui1 : spspowerguiLib/powergui  Priority=1  SimulationMode=Discrete  SampleTime=1e-6  frequency=60  Iterations=50  frequencyindice=50  Pbase=100e6  ErrMax=1e-4  UnitsV=kV  UnitsW=MW  buscounter=0  FunctionMessages=off  echomessages=off  EnableUseOfTLC=off  CurrentSourceSwitches=off  DisableSnubberDevices=off  DisableRonSwitches=off  DisableVfSwitches=off  DisplayEquations=off  AutomaticDiscreteSolvers=off  SolverType=Tustin/Backward Euler (TBE)  Interpol=off  ExternalGateDelay=off  methode=off  Ts=100  x0status=blocks  SPID=on  SwTol=0  HookPort=off  NonlinearTolerance=1e-4  nMaxIteration=100  ContinueOnMaxIteration=off  RestoreLinks=warning  ResistiveCurrentMeasurement=off  Frange=[0:2:500]  Ylog=off  Xlog=on  ShowGrid=off  save=off  variable=ZData  structure=0  ZoomFFT=off  StartTime=0.0  cycles=1  DisplayStyle=1  fundamental=60  FreqAxis=off  MaxFrequency=1000  frequencyindicesteady=1  RmsSteady=1  display=off
  powergui2 : spspowerguiLib/powergui  Priority=1  SimulationMode=Discrete  SampleTime=1e-6  frequency=60  Iterations=50  frequencyindice=50  Pbase=100e6  ErrMax=1e-4  UnitsV=kV  UnitsW=MW  buscounter=0  FunctionMessages=off  echomessages=off  EnableUseOfTLC=off  CurrentSourceSwitches=off  DisableSnubberDevices=off  DisableRonSwitches=off  DisableVfSwitches=off  DisplayEquations=off  AutomaticDiscreteSolvers=off  SolverType=Tustin/Backward Euler (TBE)  Interpol=off  ExternalGateDelay=off  methode=off  Ts=100  x0status=blocks  SPID=on  SwTol=0  HookPort=off  NonlinearTolerance=1e-4  nMaxIteration=100  ContinueOnMaxIteration=off  RestoreLinks=warning  ResistiveCurrentMeasurement=off  Frange=[0:2:500]  Ylog=off  Xlog=on  ShowGrid=off  save=off  variable=ZData  structure=0  ZoomFFT=off  StartTime=0.0  cycles=1  DisplayStyle=1  fundamental=60  FreqAxis=off  MaxFrequency=1000  frequencyindicesteady=1  RmsSteady=1  display=off
  wires:
  Constant1/1 -> PV Array/2
  Constant/1 -> PV Array/1
  VDC/1 -> [VDC1]
  [PWM11] -> Mosfet/1
  [PWM31] -> Mosfet1/1
  [PWM21] -> Mosfet2/1
  [PWM41] -> Mosfet3/1
  Current Measurement/1 -> [Igrid1]
  Voltage Measurement/1 -> [Vgrid1]
  [Vgrid1] -> [Beta1], First-Order Filter/1
  First-Order Filter/1 -> First-Order Filter1/1
  First-Order Filter1/1 -> Gain/1
  Gain/1 -> [Alpha1]
  [Alpha1] -> Mux/1
  [Beta1] -> Mux/2
  Constant2/1 -> Mux/3
  Mux/1 -> Alpha-Beta-Zero to dq0/1
  Alpha-Beta-Zero to dq0/1 -> Demux/1
  Demux/2 -> Sum/2
  Constant3/1 -> Sum/1
  Sum/1 -> PID Controller/1
  PID Controller/1 -> Integrator/1
  Integrator/1 -> MATLAB Function/1(u), Alpha-Beta-Zero to dq0/2, MATLAB Function1/1(u)
  MATLAB Function/1(y) -> [coswt1]
  PV Array/1 -> Bus Selector/1
  Unit Delay1/1 -> MATLAB Function2/2(I), Cold Weather/2
  Unit Delay/1 -> Sum1/2, Cold Weather/1, MATLAB Function2/1(V)
  MATLAB Function2/1(Vref) -> Sum1/1
  Sum1/1 -> PID Controller1/1
  PID Controller1/1 -> Sum2/1
  Gain1/1 -> Sum2/2
  Cold Weather/1 -> [Power1]
  [Power1] -> Gain1/1
  Sum2/1 -> Product1/1
  MATLAB Function1/1(y) -> [sinwt1]
  [coswt1] -> Product1/2
  Product1/1 -> Sum3/1
  IDC/1 -> [Iinv1]
  [Iinv1] -> Sum3/2
  Sum3/1 -> Sum4/1, Gain3/1
  Sum4/1 -> Gain2/1
  Gain2/1 -> Integrator1/1
  Integrator2/1 -> Gain4/1
  Gain4/1 -> Sum4/2
  Integrator1/1 -> Sum5/1, Integrator2/1
  Gain3/1 -> Sum5/2
  Sum5/1 -> Sum6/1
  [Vgrid1] -> Sum6/2
  Sum6/1 -> Product2/1
  [VDC1] -> Product2/2
  Gain5/1 -> Relational Operator1/1
  Product2/1 -> Gain5/1, Relational Operator/1
  Repeating Sequence/1 -> Relational Operator/2
  Repeating Sequence1/1 -> Relational Operator1/2
  Relational Operator/1 -> [PWM11], Logical Operator1/1
  Relational Operator1/1 -> Logical Operator/1, [PWM31]
  Logical Operator1/1 -> [PWM21]
  Logical Operator/1 -> [PWM41]
  Bus Selector/1 -> Unit Delay/1  "<V_PV>"
  Bus Selector/2 -> Unit Delay1/1  "<I_PV>"
  [Vgrid1] -> Scope/1
  [Igrid1] -> Scope/2
  [VDC1] -> Scope1/1
  [Power1] -> Scope1/2
  Unit Delay2/1 -> Sum8/2, Moddest Weather/1, MATLAB Function5/1(V)
  Gain7/1 -> Sum9/2
  Moddest Weather/1 -> [Power]
  Gain6/1 -> [Alpha]
  Constant7/1 -> Sum7/1
  Unit Delay3/1 -> MATLAB Function5/2(I), Moddest Weather/2
  MATLAB Function5/1(Vref) -> Sum8/1
  MATLAB Function3/1(y) -> [coswt]
  Sum7/1 -> PID Controller2/1
  PV Array1/1 -> Bus Selector1/1
  [Alpha] -> Mux1/1
  Alpha-Beta-Zero to dq1/1 -> Demux1/1
  First-Order Filter3/1 -> Gain6/1
  Current Measurement1/1 -> [Igrid]
  Voltage Measurement1/1 -> [Vgrid]
  First-Order Filter2/1 -> First-Order Filter3/1
  Constant5/1 -> PV Array1/2
  VDC1/1 -> [VDC]
  Constant6/1 -> Mux1/3
  Constant4/1 -> PV Array1/1
  [PWM4] -> Mosfet7/1
  [VDC] -> Scope3/1
  [PWM3] -> Mosfet5/1
  IDC1/1 -> [Iinv]
  [Power] -> Scope3/2
  Sum8/1 -> PID Controller3/1
  Gain11/1 -> Relational Operator3/1
  Sum11/1 -> Gain8/1
  [Igrid] -> Scope2/2
  Integrator3/1 -> MATLAB Function3/1(u), Alpha-Beta-Zero to dq1/2, MATLAB Function4/1(u)
  [PWM2] -> Mosfet6/1
  Bus Selector1/2 -> Unit Delay3/1  "<I_PV>"
  Relational Operator2/1 -> [PWM1], Logical Operator3/1
  [PWM1] -> Mosfet4/1
  Product5/1 -> Gain11/1, Relational Operator2/1
  Relational Operator3/1 -> Logical Operator2/1, [PWM3]
  Logical Operator3/1 -> [PWM2]
  MATLAB Function4/1(y) -> [sinwt]
  [VDC] -> Product5/2
  Repeating Sequence2/1 -> Relational Operator2/2
  [Vgrid] -> Scope2/1
  Mux1/1 -> Alpha-Beta-Zero to dq1/1
  Gain8/1 -> Integrator4/1
  Bus Selector1/1 -> Unit Delay2/1  "<V_PV>"
  Demux1/2 -> Sum7/2
  Sum13/1 -> Product5/1
  [Power] -> Gain7/1
  Integrator5/1 -> Gain10/1
  Sum12/1 -> Sum13/1
  Sum10/1 -> Sum11/1, Gain9/1
  [coswt] -> Product4/2
  PID Controller3/1 -> Sum9/1
  Gain9/1 -> Sum12/2
  Repeating Sequence3/1 -> Relational Operator3/2
  [Vgrid] -> [Beta], First-Order Filter2/1
  Sum9/1 -> Product4/1
  PID Controller2/1 -> Integrator3/1
  Logical Operator2/1 -> [PWM4]
  [Iinv] -> Sum10/2
  [Vgrid] -> Sum13/2
  Product4/1 -> Sum10/1
  Integrator4/1 -> Sum12/1, Integrator5/1
  Gain10/1 -> Sum11/2
  [Beta] -> Mux1/2
  [Vgrid3] -> Sum17/2
  [Iinv3] -> Sum14/2
  [Vgrid3] -> [Beta3], First-Order Filter4/1
  Integrator7/1 -> Sum16/1, Integrator8/1
  [Beta3] -> Mux2/2
  Product7/1 -> Sum14/1
  PID Controller4/1 -> Integrator6/1
  Logical Operator4/1 -> [PWM43]
  [Power3] -> Gain15/1
  Repeating Sequence5/1 -> Relational Operator5/2
  Gain17/1 -> Sum16/2
  PID Controller5/1 -> Sum20/1
  Demux2/2 -> Sum18/2
  Bus Selector2/1 -> Unit Delay4/1  "<V_PV>"
  Integrator8/1 -> Gain12/1
  Sum16/1 -> Sum17/1
  [VDC3] -> Product8/2
  Product8/1 -> Gain13/1, Relational Operator4/1
  Sum20/1 -> Product7/1
  Mux2/1 -> Alpha-Beta-Zero to dq2/1
  MATLAB Function7/1(y) -> [sinwt3]
  [Vgrid3] -> Scope4/1
  Logical Operator5/1 -> [PWM23]
  Gain16/1 -> Integrator7/1
  Bus Selector2/2 -> Unit Delay5/1  "<I_PV>"
  [PWM23] -> Mosfet10/1
  [Power3] -> Scope5/2
  IDC2/1 -> [Iinv3]
  Integrator6/1 -> MATLAB Function6/1(u), Alpha-Beta-Zero to dq2/2, MATLAB Function7/1(u)
  Gain13/1 -> Relational Operator5/1
  Sum15/1 -> Gain16/1
  Constant8/1 -> PV Array2/1
  Relational Operator5/1 -> Logical Operator4/1, [PWM33]
  Voltage Measurement2/1 -> [Vgrid3]
  [VDC3] -> Scope5/1
  [PWM33] -> Mosfet9/1
  [PWM43] -> Mosfet11/1
  Constant10/1 -> Mux2/3
  Hot Weather/1 -> [Power3]
  Current Measurement2/1 -> [Igrid3]
  Constant11/1 -> Sum18/1
  PV Array2/1 -> Bus Selector2/1
  Constant9/1 -> PV Array2/2
  Sum14/1 -> Sum15/1, Gain17/1
  Gain12/1 -> Sum15/2
  Sum18/1 -> PID Controller4/1
  MATLAB Function8/1(Vref) -> Sum19/1
  MATLAB Function6/1(y) -> [coswt3]
  Unit Delay5/1 -> MATLAB Function8/2(I), Hot Weather/2
  VDC2/1 -> [VDC3]
  Sum17/1 -> Product8/1
  [coswt3] -> Product7/2
  Unit Delay4/1 -> Sum19/2, Hot Weather/1, MATLAB Function8/1(V)
  [Alpha3] -> Mux2/1
  Gain15/1 -> Sum20/2
  Relational Operator4/1 -> [PWM13], Logical Operator5/1
  [Igrid3] -> Scope4/2
  First-Order Filter5/1 -> Gain14/1
  Alpha-Beta-Zero to dq2/1 -> Demux2/1
  First-Order Filter4/1 -> First-Order Filter5/1
  [PWM13] -> Mosfet8/1
  Repeating Sequence4/1 -> Relational Operator4/2
  Gain14/1 -> [Alpha3]
  Sum19/1 -> PID Controller5/1
  [Power3] -> Scope6/3
  [Power] -> Scope6/2
  [Power1] -> Scope6/1
  connections:
  PV Array/RConn1 -- VDC/LConn1 -- Series RLC Branch/LConn1 -- Mosfet1/LConn1 -- Mosfet/LConn1
  Series RLC Branch/RConn1 -- Voltage Measurement/LConn2 -- AC Voltage Source/LConn1 -- Series RLC Branch2/RConn1 -- Mosfet3/RConn1 -- Mosfet2/RConn1 -- VDC/LConn2 -- PV Array/RConn2
  Mosfet1/RConn1 -- Mosfet3/LConn1
  Mosfet/RConn1 -- IDC/LConn1 -- Mosfet2/LConn1
  IDC/RConn1 -- Series RLC Branch1/LConn1
  Series RLC Branch1/RConn1 -- Series RLC Branch3/LConn1 -- Series RLC Branch2/LConn1
  Current Measurement/LConn1 -- Series RLC Branch3/RConn1
  AC Voltage Source/RConn1 -- Voltage Measurement/LConn1 -- Current Measurement/RConn1
  Mosfet4/LConn1 -- Mosfet5/LConn1 -- PV Array1/RConn1 -- VDC1/LConn1 -- Series RLC Branch4/LConn1
  Current Measurement1/RConn1 -- AC Voltage Source1/RConn1 -- Voltage Measurement1/LConn1
  Mosfet6/RConn1 -- Series RLC Branch4/RConn1 -- PV Array1/RConn2 -- VDC1/LConn2 -- Voltage Measurement1/LConn2 -- AC Voltage Source1/LConn1 -- Series RLC Branch6/RConn1 -- Mosfet7/RConn1
  Series RLC Branch6/LConn1 -- Series RLC Branch5/RConn1 -- Series RLC Branch7/LConn1
  Mosfet6/LConn1 -- Mosfet4/RConn1 -- IDC1/LConn1
  Mosfet5/RConn1 -- Mosfet7/LConn1
  IDC1/RConn1 -- Series RLC Branch5/LConn1
  Current Measurement1/LConn1 -- Series RLC Branch7/RConn1
  Series RLC Branch10/LConn1 -- Series RLC Branch9/RConn1 -- Series RLC Branch11/LConn1
  Mosfet10/LConn1 -- Mosfet8/RConn1 -- IDC2/LConn1
  Mosfet10/RConn1 -- Voltage Measurement2/LConn2 -- AC Voltage Source2/LConn1 -- Series RLC Branch10/RConn1 -- Mosfet11/RConn1 -- Series RLC Branch8/RConn1 -- PV Array2/RConn2 -- VDC2/LConn2
  Series RLC Branch8/LConn1 -- PV Array2/RConn1 -- VDC2/LConn1 -- Mosfet9/LConn1 -- Mosfet8/LConn1
  Current Measurement2/RConn1 -- AC Voltage Source2/RConn1 -- Voltage Measurement2/LConn1
  Current Measurement2/LConn1 -- Series RLC Branch11/RConn1
  IDC2/RConn1 -- Series RLC Branch9/LConn1
  Mosfet9/RConn1 -- Mosfet11/LConn1

== matlab function SinglePhasePVGridConnettedArray/MATLAB Function ==
  data: u input; y output
function y = fcn(u)

y = cos(u(1));

== matlab function SinglePhasePVGridConnettedArray/MATLAB Function2 ==
  data: V input; Vref output; I input
function Vref = RefGen(V,I)

Vrefmax = 550;
Vrefmin = 0.0;
Vrefinit= 420;
deltaVref = 1;
persistent Void Poid Vrefold;

dataType = 'double';

if isempty(Void)
    Void=0;
    Poid=0;
    Vrefold=Vrefinit;
    
end
P=V*I;
dV= V - Void;
dP= P - Poid;

if dP ~= 0
    if dP < 0
        if dV < 0
            Vref = Vrefold + deltaVref;
        else
            Vref = Vrefold - deltaVref;
        end
    else
        if dV < 0
        Vref = Vrefold + deltaVref;
    else
        Vref = Vrefold + deltaVref;
    end
  end

else Vref=Vrefold;

end
if Vref >= Vrefmax || Vref<= Vrefmin
    Vref=Vrefold;
end

Vrefold=Vref;
Void=V;
Poid=P;

== matlab function SinglePhasePVGridConnettedArray/MATLAB Function3 ==
  data: u input; y output
function y = fcn(u)

y = cos(u(1));

== matlab function SinglePhasePVGridConnettedArray/MATLAB Function4 ==
  data: u input; y output
function y = fcn(u)

y = sin(u(1));

== matlab function SinglePhasePVGridConnettedArray/MATLAB Function5 ==
  data: V input; Vref output; I input
function Vref = RefGen(V,I)

Vrefmax = 550;
Vrefmin = 0.0;
Vrefinit= 420;
deltaVref = 1;
persistent Void Poid Vrefold;

dataType = 'double';

if isempty(Void)
    Void=0;
    Poid=0;
    Vrefold=Vrefinit;
    
end
P=V*I;
dV= V - Void;
dP= P - Poid;

if dP ~= 0
    if dP < 0
        if dV < 0
            Vref = Vrefold + deltaVref;
        else
            Vref = Vrefold - deltaVref;
        end
    else
        if dV < 0
        Vref = Vrefold + deltaVref;
    else
        Vref = Vrefold + deltaVref;
    end
  end

else Vref=Vrefold;

end
if Vref >= Vrefmax || Vref<= Vrefmin
    Vref=Vrefold;
end

Vrefold=Vref;
Void=V;
Poid=P;

== matlab function SinglePhasePVGridConnettedArray/MATLAB Function6 ==
  data: u input; y output
function y = fcn(u)

y = cos(u(1));

== matlab function SinglePhasePVGridConnettedArray/MATLAB Function7 ==
  data: u input; y output
function y = fcn(u)

y = sin(u(1));

== matlab function SinglePhasePVGridConnettedArray/MATLAB Function8 ==
  data: V input; Vref output; I input
function Vref = RefGen(V,I)

Vrefmax = 550;
Vrefmin = 0.0;
Vrefinit= 420;
deltaVref = 1;
persistent Void Poid Vrefold;

dataType = 'double';

if isempty(Void)
    Void=0;
    Poid=0;
    Vrefold=Vrefinit;
    
end
P=V*I;
dV= V - Void;
dP= P - Poid;

if dP ~= 0
    if dP < 0
        if dV < 0
            Vref = Vrefold + deltaVref;
        else
            Vref = Vrefold - deltaVref;
        end
    else
        if dV < 0
        Vref = Vrefold + deltaVref;
    else
        Vref = Vrefold + deltaVref;
    end
  end

else Vref=Vrefold;

end
if Vref >= Vrefmax || Vref<= Vrefmin
    Vref=Vrefold;
end

Vrefold=Vref;
Void=V;
Poid=P;

== matlab function SinglePhasePVGridConnettedArray/MATLAB Function1 ==
  data: u input; y output
function y = fcn(u)

y = sin(u(1));
